simulink model "q_ip02_speed_pi"  (Simulink 10.3)
settings: Solver=ode4  StartTime=0.0  StopTime=inf  FixedStep=0.001  RelTol=1e-3  AbsTol=1e-6  EnableMultiTasking=on
values from neighbouring files (symbols this model uses):
  bsp = 0    [setup_ip02_speed.m]
  K = 0.1    [setup_ip02_speed.m]
  K_AMP = 1    [setup_ip02_speed.m]
  ki = 0    [setup_ip02_speed.m]
  kp = 0    [setup_ip02_speed.m]
  tau = 0.01    [setup_ip02_speed.m]
  VMAX_DAC = 10    [setup_ip02_speed.m]
  wcf = 2 * pi * 70    (= 439.822971503)    [setup_ip02_speed.m]
  X_LIM_ENABLE = 1    [setup_ip02_speed.m]
  X_MAX = 0.35    [setup_ip02_speed.m]
  X_MIN = - X_MAX    (= -0.35)    [setup_ip02_speed.m]
  zetaf = 0.9    [setup_ip02_speed.m]
undefined symbols (not defined in the file or in its folder): HIL, K_EC, K_EP, qc_get_step_size, VMAX_AMP
libraries: quarc_library x5, simulink_extras x1
settings Model: Creator=Mfotoohi  LastModifiedBy=MLevis  SimulationMode=external  ExtModeTrigDuration=10000
settings SolverCC: AutoScaleAbsTol=off  PositivePriorityOrder=on
settings OptimizationCC: BooleanDataType=off  OptimizeBlockIOStorage=off  BufferReuse=off  ExpressionFolding=off  LocalBlockOutputs=off  InitFltsAndDblsToZero=on  LifeSpan=auto
settings DebuggingCC: SaveWithParameterizedLinksMsg=none  SignalResolutionControl=TryResolveAllWithWarning  MultiTaskDSMMsg=warning  MultiTaskCondExecSysMsg=none
settings HardwareCC: ProdBitPerPointer=64  ProdBitPerSizeT=64  ProdBitPerPtrDiffT=64  ProdLargestAtomicFloat=Float  ProdIntDivRoundTo=Zero  ProdEndianess=LittleEndian  ProdWordSize=64  ProdHWDeviceType=Intel->x86-64 (Windows64)  TargetHWDeviceType=32-bit Generic
settings RTWCC: Description=QUARC Win64 Target Using Toolchain  SystemTargetFile=quarc_win64.tlc  TemplateMakefile=quarc_default_tmf  Toolchain=QUARC win64 | nmake (64-bit Windows)  BuildConfiguration=Faster Runs
settings STFCustomTargetCC: ConcurrentExecutionCompliant=on  UseToolchainInfoCompliant=on  SystemTargetFile=quarc_win64.tlc
settings GRTTargetCC: ParMdlRefBuildCompliant=off  CompOptLevelCompliant=off  MatFileLogging=off  CPPClassGenCompliant=off  ExtMode=on  ExtModeMexFile=quarc_comm

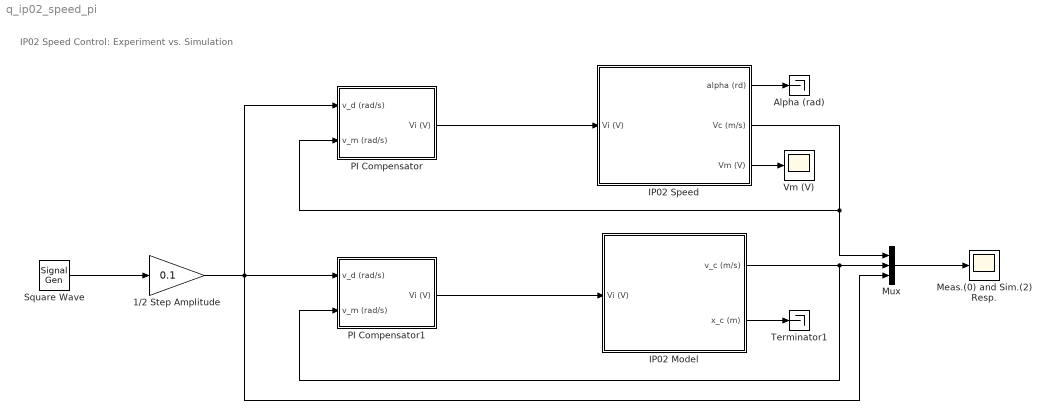
== system q_ip02_speed_pi ==
  note: IP02 Speed Control:
      | Experiment vs. Simulation
  1/2 Step Amplitude : Gain  Gain=0.1  SaturateOnIntegerOverflow=on  OutDataTypeStr=Inherit: Same as input  ParamDataTypeStr=Inherit: Same as input
  Alpha (rad) : Terminator
  IP02 Model : Subsystem
  IP02 Speed : Subsystem
  Meas.(0) and Sim.(2) Resp. : Scope
  Mux : Mux  Inputs=3
  PI Compensator : Subsystem
  PI Compensator1 : Subsystem
  Square Wave : SignalGenerator  WaveForm=square  Frequency=0.3
  Terminator1 : Terminator
  Vm (V) : Scope
  wires:
  Mux/1 -> Meas.(0) and Sim.(2) Resp./1
  1/2 Step Amplitude/1 -> PI Compensator1/1(v_d (rad/s)), Mux/3, PI Compensator/1(v_d (rad/s))
  IP02 Speed/2(Vc (m/s)) -> Mux/1, PI Compensator/2(v_m (rad/s))
  IP02 Model/1(v_c (m/s)) -> Mux/2, PI Compensator1/2(v_m (rad/s))
  IP02 Model/2(x_c (m)) -> Terminator1/1
  PI Compensator/1(Vi (V)) -> IP02 Speed/1(Vi (V))
  IP02 Speed/1(alpha (rd)) -> Alpha (rad)/1
  IP02 Speed/3(Vm (V)) -> Vm (V)/1
  PI Compensator1/1(Vi (V)) -> IP02 Model/1(Vi (V))
  Square Wave/1 -> 1/2 Step Amplitude/1

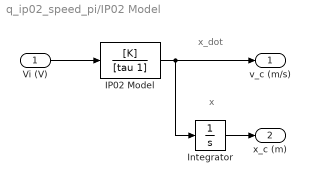
== system q_ip02_speed_pi/IP02 Model ==
  note: x_dot
  note: x
  Vi (V) : Inport
  IP02 Model : TransferFcn  Numerator=[K]  Denominator=[tau 1]
  Integrator : Integrator
  v_c (m/s) : Outport
  x_c (m) : Outport  Port=2
  wires:
  IP02 Model/1 -> v_c (m/s)/1, Integrator/1
  Vi (V)/1 -> IP02 Model/1
  Integrator/1 -> x_c (m)/1

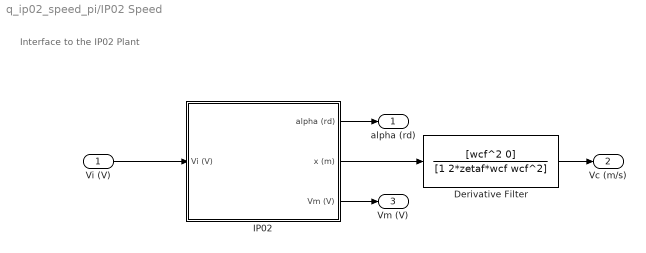
== system q_ip02_speed_pi/IP02 Speed ==
  note: Interface to the IP02 Plant
  Vi (V) : Inport
  Derivative Filter : TransferFcn  Numerator=[wcf^2 0]  Denominator=[1 2*zetaf*wcf wcf^2]
  IP02 : Subsystem
  alpha (rd) : Outport  InitialOutput=0
  Vc (m/s) : Outport  Port=2  InitialOutput=0
  Vm (V) : Outport  Port=3  InitialOutput=0
  wires:
  IP02/3(Vm (V)) -> Vm (V)/1
  Vi (V)/1 -> IP02/1(Vi (V))
  IP02/1(alpha (rd)) -> alpha (rd)/1
  IP02/2(x (m)) -> Derivative Filter/1
  Derivative Filter/1 -> Vc (m/s)/1

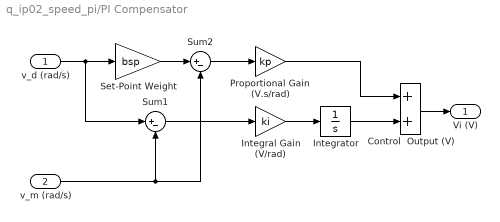
== system q_ip02_speed_pi/PI Compensator ==
  v_d (rad/s) : Inport
  v_m (rad/s) : Inport  Port=2
  Control  Output (V) : Sum
  Integral Gain (V/rad) : Gain  Gain=ki
  Integrator : Integrator  UpperSaturationLimit=10  LowerSaturationLimit=-10
  Proportional Gain  (V.s/rad) : Gain  Gain=kp
  Set-Point Weight : Gain  Gain=bsp
  Sum1 : Sum  Inputs=|+-
  Sum2 : Sum  Inputs=|+-
  Vi (V) : Outport
  wires:
  v_m (rad/s)/1 -> Sum2/2, Sum1/2
  Control  Output (V)/1 -> Vi (V)/1
  v_d (rad/s)/1 -> Sum1/1, Set-Point Weight/1
  Sum2/1 -> Proportional Gain  (V.s/rad)/1
  Set-Point Weight/1 -> Sum2/1
  Proportional Gain  (V.s/rad)/1 -> Control  Output (V)/1
  Integral Gain (V/rad)/1 -> Integrator/1
  Sum1/1 -> Integral Gain (V/rad)/1
  Integrator/1 -> Control  Output (V)/2

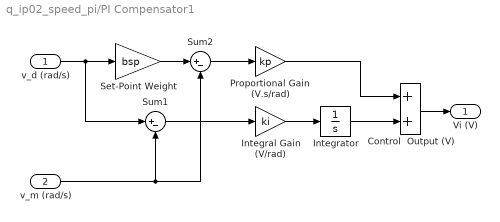
== system q_ip02_speed_pi/PI Compensator1 ==
  v_d (rad/s) : Inport
  v_m (rad/s) : Inport  Port=2
  Control  Output (V) : Sum
  Integral Gain (V/rad) : Gain  Gain=ki
  Integrator : Integrator  UpperSaturationLimit=10  LowerSaturationLimit=-10
  Proportional Gain  (V.s/rad) : Gain  Gain=kp
  Set-Point Weight : Gain  Gain=bsp
  Sum1 : Sum  Inputs=|+-
  Sum2 : Sum  Inputs=|+-
  Vi (V) : Outport
  wires:
  Sum1/1 -> Integral Gain (V/rad)/1
  Integral Gain (V/rad)/1 -> Integrator/1
  Integrator/1 -> Control  Output (V)/2
  Proportional Gain  (V.s/rad)/1 -> Control  Output (V)/1
  Set-Point Weight/1 -> Sum2/1
  Sum2/1 -> Proportional Gain  (V.s/rad)/1
  v_d (rad/s)/1 -> Set-Point Weight/1, Sum1/1
  Control  Output (V)/1 -> Vi (V)/1
  v_m (rad/s)/1 -> Sum1/2, Sum2/2

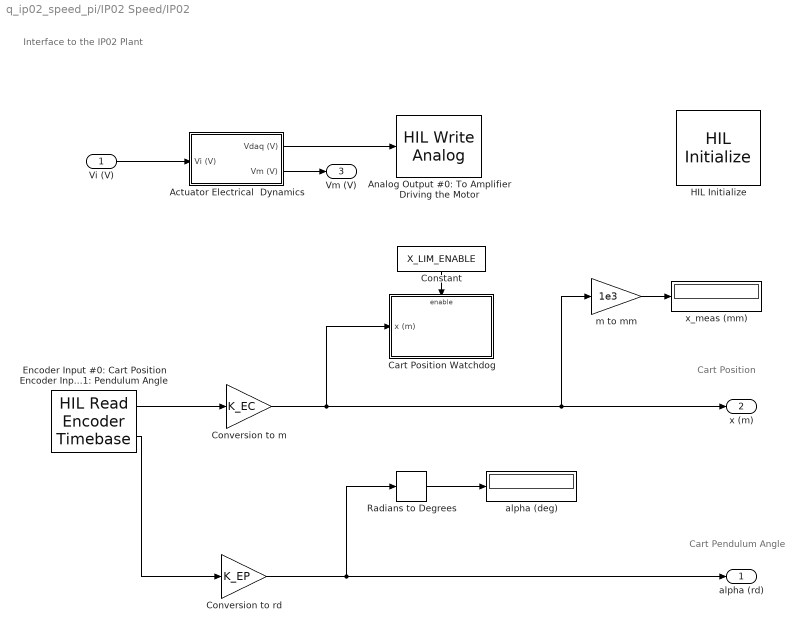
== system q_ip02_speed_pi/IP02 Speed/IP02 ==
  note: Cart Pendulum Angle
  note: Cart Position
  note: Interface to the IP02 Plant
  Vi (V) : Inport
  Actuator Electrical  Dynamics : Subsystem
  Analog Output #0: To Amplifier Driving the Motor : quarc_library/Data Acquisition/Generic/Immediate I//O/HIL Write Analog  Tag=unassigned  object_name=HIL-1  channels=0  sample_time=-1  active=on  vector_input=on
  Cart Position Watchdog : Subsystem  TreatAsAtomicUnit=on
  Constant : Constant  Value=X_LIM_ENABLE
  Conversion to m : Gain  Gain=K_EC  SaturateOnIntegerOverflow=on  OutDataTypeStr=Inherit: Same as input  ParamDataTypeStr=Inherit: Same as input
  Conversion to rd : Gain  Gain=K_EP  SaturateOnIntegerOverflow=on  OutDataTypeStr=Inherit: Same as input  ParamDataTypeStr=Inherit: Same as input
  Encoder Input #0: Cart Position Encoder Input #1: Pendulum Angle : quarc_library/Data Acquisition/Generic/Timebases/HIL Read Encoder Timebase  Tag=unassigned  object_name=HIL-1  clock=0  channels=[0,1]  active=on  vector_output=off  data_type_mode=Inherit via back propagation  data_type=double  overflow_mode=Error on overflow  samples_in_buffer=max(ceil(1/qc_get_step_size), 1)
  HIL Initialize : quarc_library/Data Acquisition/Generic/Configuration/HIL Initialize  object_name=HIL-1  board_type=q2_usb  board_number=0  board_options=d0=digital;d1=digital;led=auto;update_rate=normal  exclusive=off  active=off  hardware_clocks=[0:2]  clock_modes=[]  initial_clock_frequencies=[]  set_clock_params_at_start=off  set_clock_params_at_switch_in=off  set_clock_frequencies_at_start=off  set_clock_frequencies_at_switch_in=off  analog_input_channels=[0:1]  analog_input_configurations=[]  analog_input_maximums=10  analog_input_minimums=-10  set_analog_input_params_at_start=on  set_analog_input_params_at_switch_in=off  analog_output_channels=[0:1]  analog_output_maximums=10  analog_output_minimums=-10  initial_analog_outputs=[0]  final_analog_outputs=[0]  watchdog_analog_outputs=0  set_analog_output_params_at_start=on  set_analog_output_params_at_switch_in=off  set_analog_outputs_at_start=on  set_analog_outputs_at_switch_in=off  set_analog_outputs_at_terminate=on  set_analog_outputs_at_switch_out=off  set_analog_outputs_on_watchdog=off  digital_input_channels=[]  digital_output_channels=[0:7]  digital_output_configuration=[]  initial_digital_outputs=[0]  final_digital_outputs=[0]  watchdog_digital_outputs=[0]  set_digital_output_params_at_start=off  set_digital_output_params_at_switch_in=off  set_digital_outputs_at_start=on  set_digital_outputs_at_switch_in=off  set_digital_outputs_at_terminate=on  set_digital_outputs_at_switch_out=off  set_digital_outputs_on_watchdog=off  encoder_channels=[0:1]  quadrature=[4]  encoder_filter_frequency=[]  initial_encoder_counts=[0]  set_encoder_params_at_start=on  set_encoder_params_at_switch_in=off  set_encoder_counts_at_start=on  set_encoder_counts_at_switch_in=off  pwm_channels=[]  pwm_modes=[0]  pwm_frequency=1/0.020  pwm_configuration=[]  pwm_alignment=[]  pwm_polarity=[]  pwm_leading_deadband=[]  pwm_trailing_deadband=[]  initial_pwm_outputs=[0]  final_pwm_outputs=[0]  watchdog_pwm_outputs=[0]  set_pwm_params_at_start=on  set_pwm_params_at_switch_in=off  set_pwm_outputs_at_start=on  set_pwm_outputs_at_switch_in=off  set_pwm_outputs_at_terminate=on  set_pwm_outputs_at_switch_out=off  set_pwm_outputs_on_watchdog=off  other_output_channels=[]  initial_other_outputs=[]  final_other_outputs=[]  watchdog_other_outputs=[]  set_other_outputs_at_start=off  set_other_outputs_at_switch_in=off  set_other_outputs_at_terminate=off  set_other_outputs_at_switch_out=off  set_other_outputs_on_watchdog=off
  Radians to Degrees : simulink_extras/Transformations/Radians to Degrees
  alpha (deg) : Display
      settings: Decimation=100
  m to mm : Gain  Gain=1e3  SaturateOnIntegerOverflow=on  OutDataTypeStr=Inherit: Same as input  ParamDataTypeStr=Inherit: Same as input
  x_meas (mm) : Display
      settings: Decimation=100
  alpha (rd) : Outport  InitialOutput=0
  x (m) : Outport  Port=2  InitialOutput=0
  Vm (V) : Outport  Port=3  InitialOutput=0
  wires:
  Encoder Input #0: Cart Position Encoder Input #1: Pendulum Angle/1 -> Conversion to m/1
  Conversion to m/1 -> Cart Position Watchdog/1(x (m)), x (m)/1, m to mm/1
  m to mm/1 -> x_meas (mm)/1
  Encoder Input #0: Cart Position Encoder Input #1: Pendulum Angle/2 -> Conversion to rd/1
  Radians to Degrees/1 -> alpha (deg)/1
  Conversion to rd/1 -> Radians to Degrees/1, alpha (rd)/1
  Constant/1 -> Cart Position Watchdog/Enable
  Actuator Electrical  Dynamics/1(Vdaq (V)) -> Analog Output #0: To Amplifier Driving the Motor/1
  Vi (V)/1 -> Actuator Electrical  Dynamics/1(Vi (V))
  Actuator Electrical  Dynamics/2(Vm (V)) -> Vm (V)/1

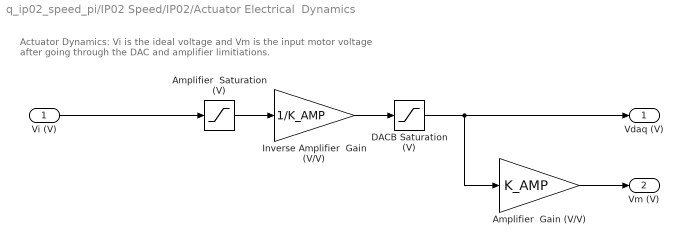
== system q_ip02_speed_pi/IP02 Speed/IP02/Actuator Electrical  Dynamics ==
  note: Actuator Dynamics: Vi is the ideal voltage and Vm is the
      | input motor voltage after going through the DAC and amplifier limitiations.
  Vi (V) : Inport
  Amplifier  Gain (V/V) : Gain  Gain=K_AMP
  Amplifier  Saturation (V) : Saturate  UpperLimit=VMAX_AMP  LowerLimit=-VMAX_AMP
  DACB Saturation (V) : Saturate  UpperLimit=VMAX_DAC  LowerLimit=-VMAX_DAC
  Inverse Amplifier  Gain (V/V) : Gain  Gain=1/K_AMP
  Vdaq (V) : Outport
  Vm (V) : Outport  Port=2
  wires:
  Vi (V)/1 -> Amplifier  Saturation (V)/1
  Amplifier  Saturation (V)/1 -> Inverse Amplifier  Gain (V/V)/1
  Inverse Amplifier  Gain (V/V)/1 -> DACB Saturation (V)/1
  DACB Saturation (V)/1 -> Amplifier  Gain (V/V)/1, Vdaq (V)/1
  Amplifier  Gain (V/V)/1 -> Vm (V)/1

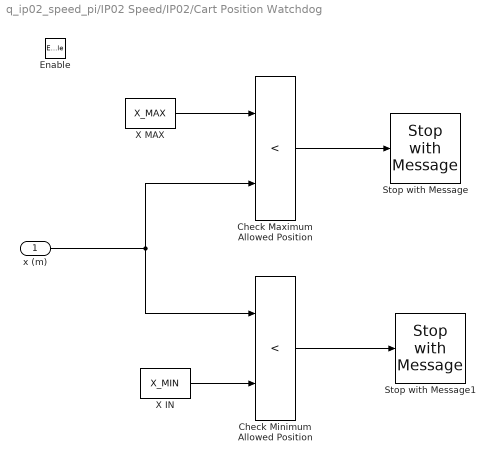
== system q_ip02_speed_pi/IP02 Speed/IP02/Cart Position Watchdog ==
  x (m) : Inport
  Enable : EnablePort
  Check Maximum Allowed Position : RelationalOperator  Operator=<  RndMeth=Nearest  InputSameDT=on
  Check Minimum Allowed Position : RelationalOperator  Operator=<  RndMeth=Nearest  InputSameDT=on
  Stop with Message : quarc_library/Sinks/Error Handling/Stop with Message  message_type=Fixed error message  message_icon=Error  message=Maximum Limit Reached.
  Stop with Message1 : quarc_library/Sinks/Error Handling/Stop with Message  message_type=Fixed error message  message_icon=Error  message=Minimum Limit Reached.
  X IN : Constant  Value=X_MIN
  X MAX : Constant  Value=X_MAX
  wires:
  Check Maximum Allowed Position/1 -> Stop with Message/1
  x (m)/1 -> Check Minimum Allowed Position/1, Check Maximum Allowed Position/2
  X IN/1 -> Check Minimum Allowed Position/2
  Check Minimum Allowed Position/1 -> Stop with Message1/1
  X MAX/1 -> Check Maximum Allowed Position/1
